simulink model "IEEE_39_IBR_Simplified"  (R2023b)
settings: Solver=FixedStepAuto  StartTime=0  StopTime=20  FixedStep=Ts  MaxStep=1/60  RelTol=1e-3  AbsTol=1e-2  EnableMultiTasking=on
PreLoadFcn:
  | NE39bus_data;
  | PSSMODEL=1;
  | LPSS=0;
  | WAPSS=0;
  | WAPSS2=0;
values from neighbouring files (symbols this model uses):
  Dt = 0    [SG_para.m]
  dw0_sm = 0    [SG_para.m]
  Emax = 1    [SG_para.m]
  Emin = 0.5    [SG_para.m]
  Fg = [0.1,0.1,0.1]    [SG_para.m]
  fn_sm = 60*ones(1,10)    [SG_para.m]
  H_sm = [5,3.03,3.58,2.86,2.6,3.48,2.64,2.43,3.45,4.2]*10    [SG_para.m]
  ia0_sm = 0.75*0    (= 0)    [SG_para.m]
  ib0_sm = 0.75*0    (= 0)    [SG_para.m]
  ic0_sm = 0.75*0    (= 0)    [SG_para.m]
  Kd_sm = 6*ones(1,10)    [SG_para.m]
  Ke = 200    [SG_para.m]
  Kg = [0.95,0.95,0.95]    [SG_para.m]
  Ks = 2    [SG_para.m]
  line = [     1	2	0.0035	0.0411	0.6987	0	100	345 ... (first row only)    [SG_para.m]
  p = 1    [SG_para.m]
  pha0_sm = -24.95*0    (= 0)    [SG_para.m]
  phb0_sm = -144.94*0    (= 0)    [SG_para.m]
  phc0_sm = 95.05*0    (= 0)    [SG_para.m]
  Pn_sm = [1000,1000,1000,1000,1000,1000,1000,1000,1000,1000]    [SG_para.m]
  Pref_sm = [1000 520.81 650 632 508 650 560 540 830 250]./Pn_sm    [SG_para.m]
  R = 1e-3    (= 0.001)    [SG_para.m]
  Rg = [0.05,0.05,0.05]    [SG_para.m]
  rs = 2.8544e-3    (= 0.0028544)    [SG_para.m]
  s = 1    [SG_para.m]
  s1 = 10    [SG_para.m]
  T1 = 0.05    [SG_para.m]
  T2 = 0.5    [SG_para.m]
  T3 = 0.5    [SG_para.m]
  Te = 0.05    [SG_para.m]
  Tfa = 3    [SG_para.m]
  Tfb = 10    [SG_para.m]
  Tg = [10,10,10]    [SG_para.m]
  theta0_sm = -94.3*0    (= 0)    [SG_para.m]
  Ts = 5e-5    (= 5e-05)    [SG_para.m]
  Ts1 = 0.18    [SG_para.m]
  Ts2 = 2    [SG_para.m]
  Ts3 = 5    [SG_para.m]
  Ts4 = 10    [SG_para.m]
  Ts5 = 15    [SG_para.m]
  Un_sm = [345,22,22,22,22,22,22,22,345,22]    [SG_para.m]
  Vmax = inf    [SG_para.m]
  Vmin = 0    [SG_para.m]
  Vref_sm = 1*ones(1,10)    [SG_para.m]
  xd = xd_t    (= 0.296)    [SG_para.m]
undefined symbols (not defined in the file or in its folder): D1, D11, Delta, Ka, Kf, Ta, Tf
libraries: spsThreePhaseVIMeasurementLib x41, spsThreePhaseFaultLib x39, spsThreePhaseSeriesRLCBranchLib x36, spsThreePhaseParallelRLCLoadLib x20, spsThreePhaseTransformerTwoWindingsLib x13, spsSimplifiedSynchronousMachinepuUnitsLib x10, spsLoadFlowBusLib x10, Inverter_based_Resources_IBRs x10, spsThreePhaseBreakerLib x2, spsSequenceAnalyzerLib x2, spsMultimeterLib x1, eePowerMeasurement x1
(part 3 of 5)

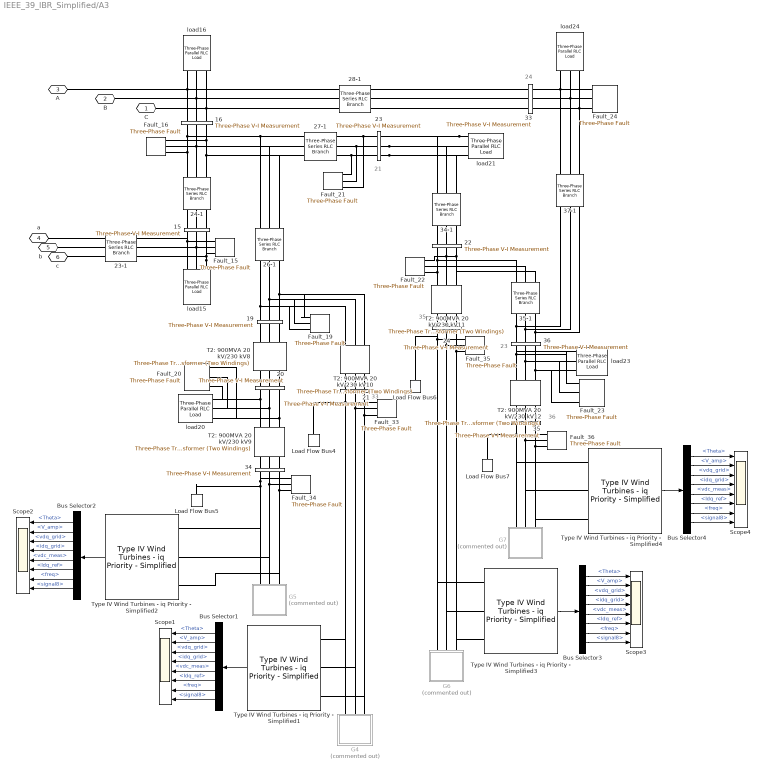
== system IEEE_39_IBR_Simplified/A3 ==
  note: 35
  note: 33
  note: 21
  note: 24
  note: 36
  note: 23
  15 : spsThreePhaseVIMeasurementLib/Three-Phase V-I Measurement  VoltageMeasurement=phase-to-phase  SetLabelV=on  LabelV=Vabc_15  Vpu=off  VpuLL=on  CurrentMeasurement=no  SetLabelI=on  LabelI=Iabc_B2  Ipu=off  Pbase=100e6  Vbase=Bus(15,2)*1e3  OutputType=Complex  PhasorSimulation=off  PSBequivalent=0
  16 : spsThreePhaseVIMeasurementLib/Three-Phase V-I Measurement  VoltageMeasurement=phase-to-phase  SetLabelV=on  LabelV=Vabc_16  Vpu=off  VpuLL=on  CurrentMeasurement=no  SetLabelI=on  LabelI=Iabc_B2  Ipu=off  Pbase=100e6  Vbase=Bus(16,2)*1e3  OutputType=Complex  PhasorSimulation=off  PSBequivalent=0
  19 : spsThreePhaseVIMeasurementLib/Three-Phase V-I Measurement  VoltageMeasurement=phase-to-phase  SetLabelV=on  LabelV=Vabc_19  Vpu=off  VpuLL=on  CurrentMeasurement=no  SetLabelI=on  LabelI=Iabc_B2  Ipu=off  Pbase=100e6  Vbase=Bus(19,2)*1e3  OutputType=Complex  PhasorSimulation=off  PSBequivalent=0
  20 : spsThreePhaseVIMeasurementLib/Three-Phase V-I Measurement  VoltageMeasurement=phase-to-phase  SetLabelV=on  LabelV=Vabc_20  Vpu=off  VpuLL=on  CurrentMeasurement=no  SetLabelI=on  LabelI=Iabc_B2  Ipu=off  Pbase=100e6  Vbase=Bus(20,2)*1e3  OutputType=Complex  PhasorSimulation=off  PSBequivalent=0
  21 : spsThreePhaseVIMeasurementLib/Three-Phase V-I Measurement  VoltageMeasurement=phase-to-phase  SetLabelV=on  LabelV=Vabc_33  Vpu=off  VpuLL=on  CurrentMeasurement=no  SetLabelI=on  LabelI=Iabc_B2  Ipu=off  Pbase=100e6  Vbase=Bus(33,2)*1e3  OutputType=Complex  PhasorSimulation=off  PSBequivalent=0
  22 : spsThreePhaseVIMeasurementLib/Three-Phase V-I Measurement  VoltageMeasurement=phase-to-phase  SetLabelV=on  LabelV=Vabc_22  Vpu=off  VpuLL=on  CurrentMeasurement=no  SetLabelI=on  LabelI=Iabc_B2  Ipu=off  Pbase=100e6  Vbase=Bus(22,2)*1e3  OutputType=Complex  PhasorSimulation=off  PSBequivalent=0
  23 : spsThreePhaseVIMeasurementLib/Three-Phase V-I Measurement  VoltageMeasurement=phase-to-phase  SetLabelV=on  LabelV=Vabc_21  Vpu=off  VpuLL=on  CurrentMeasurement=no  SetLabelI=on  LabelI=Iabc_B2  Ipu=off  Pbase=100e6  Vbase=Bus(21,2)*1e3  OutputType=Complex  PhasorSimulation=off  PSBequivalent=0
  23-1 : spsThreePhaseSeriesRLCBranchLib/Three-Phase Series RLC Branch  LConnTagsString=A|B|C  RConnTagsString=A|B|C  BranchType=RL  Resistance=line(23,3)  Inductance=line(23,4)  Capacitance=1e-6  Measurements=None
  24 : spsThreePhaseVIMeasurementLib/Three-Phase V-I Measurement  VoltageMeasurement=phase-to-phase  SetLabelV=on  LabelV=Vabc_35  Vpu=off  VpuLL=on  CurrentMeasurement=no  SetLabelI=on  LabelI=Iabc_B2  Ipu=off  Pbase=100e6  Vbase=Bus(35,2)*1e3  OutputType=Complex  PhasorSimulation=off  PSBequivalent=0
  24-1 : spsThreePhaseSeriesRLCBranchLib/Three-Phase Series RLC Branch  LConnTagsString=A|B|C  RConnTagsString=A|B|C  BranchType=RL  Resistance=line(24,3)  Inductance=line(24,4)  Capacitance=1e-6  Measurements=None
  26-1 : spsThreePhaseSeriesRLCBranchLib/Three-Phase Series RLC Branch  LConnTagsString=A|B|C  RConnTagsString=A|B|C  BranchType=RL  Resistance=line(26,3)  Inductance=line(26,4)  Capacitance=1e-6  Measurements=None
  27-1 : spsThreePhaseSeriesRLCBranchLib/Three-Phase Series RLC Branch  LConnTagsString=A|B|C  RConnTagsString=A|B|C  BranchType=RL  Resistance=line(27,3)  Inductance=line(27,4)  Capacitance=1e-6  Measurements=None
  28-1 : spsThreePhaseSeriesRLCBranchLib/Three-Phase Series RLC Branch  LConnTagsString=A|B|C  RConnTagsString=A|B|C  BranchType=RL  Resistance=line(28,3)  Inductance=line(28,4)  Capacitance=1e-6  Measurements=None
  33 : spsThreePhaseVIMeasurementLib/Three-Phase V-I Measurement  VoltageMeasurement=phase-to-phase  SetLabelV=on  LabelV=Vabc_24  Vpu=off  VpuLL=on  CurrentMeasurement=no  SetLabelI=on  LabelI=Iabc_B2  Ipu=off  Pbase=100e6  Vbase=Bus(24,2)*1e3  OutputType=Complex  PhasorSimulation=off  PSBequivalent=0
  34 : spsThreePhaseVIMeasurementLib/Three-Phase V-I Measurement  VoltageMeasurement=phase-to-phase  SetLabelV=on  LabelV=Vabc_34  Vpu=off  VpuLL=on  CurrentMeasurement=no  SetLabelI=on  LabelI=Iabc_B2  Ipu=off  Pbase=100e6  Vbase=Bus(34,2)*1e3  OutputType=Complex  PhasorSimulation=off  PSBequivalent=0
  34-1 : spsThreePhaseSeriesRLCBranchLib/Three-Phase Series RLC Branch  LConnTagsString=A|B|C  RConnTagsString=A|B|C  BranchType=RL  Resistance=line(34,3)  Inductance=line(34,4)  Capacitance=1e-6  Measurements=None
  35 : spsThreePhaseVIMeasurementLib/Three-Phase V-I Measurement  VoltageMeasurement=phase-to-phase  SetLabelV=on  LabelV=Vabc_36  Vpu=off  VpuLL=on  CurrentMeasurement=no  SetLabelI=on  LabelI=Iabc_B2  Ipu=off  Pbase=100e6  Vbase=Bus(36,2)*1e3  OutputType=Complex  PhasorSimulation=off  PSBequivalent=0
  35-1 : spsThreePhaseSeriesRLCBranchLib/Three-Phase Series RLC Branch  LConnTagsString=A|B|C  RConnTagsString=A|B|C  BranchType=RL  Resistance=line(35,3)  Inductance=line(35,4)  Capacitance=1e-6  Measurements=None
  36 : spsThreePhaseVIMeasurementLib/Three-Phase V-I Measurement  VoltageMeasurement=phase-to-phase  SetLabelV=on  LabelV=Vabc_23  Vpu=off  VpuLL=on  CurrentMeasurement=no  SetLabelI=on  LabelI=Iabc_B2  Ipu=off  Pbase=100e6  Vbase=Bus(23,2)*1e3  OutputType=Complex  PhasorSimulation=off  PSBequivalent=0
  37-1 : spsThreePhaseSeriesRLCBranchLib/Three-Phase Series RLC Branch  LConnTagsString=A|B|C  RConnTagsString=A|B|C  BranchType=RL  Resistance=line(37,3)  Inductance=line(37,4)  Capacitance=1e-6  Measurements=None
  Bus Selector{1..4} (4 alike) : BusSelector  OutputSignals=Theta,V_amp,vdq_grid,idq_grid,vdc_meas,Idq_ref,freq,signal8
  Fault_15 : spsThreePhaseFaultLib/Three-Phase Fault  InitialStates=0  FaultA=on  FaultB=on  FaultC=on  GroundFault=on  SwitchTimes="[t(15)+1/60  t(15)+5/60]"  External=off  SwitchStatus=NaN  FaultResistance=0.001  GroundResistance=0.01  SnubberResistance=1e6  SnubberCapacitance=inf  Measurements=Fault voltages and currents
  Fault_16 : spsThreePhaseFaultLib/Three-Phase Fault  InitialStates=0  FaultA=on  FaultB=on  FaultC=on  GroundFault=on  SwitchTimes="[t(16)+1/60  t(16)+5/60]"  External=off  SwitchStatus=NaN  FaultResistance=0.001  GroundResistance=0.01  SnubberResistance=1e6  SnubberCapacitance=inf  Measurements=Fault voltages and currents
  Fault_19 : spsThreePhaseFaultLib/Three-Phase Fault  InitialStates=0  FaultA=on  FaultB=on  FaultC=on  GroundFault=on  SwitchTimes="[t(19)+1/60  t(19)+5/60]"  External=off  SwitchStatus=NaN  FaultResistance=0.001  GroundResistance=0.01  SnubberResistance=1e6  SnubberCapacitance=inf  Measurements=Fault voltages and currents
  Fault_20 : spsThreePhaseFaultLib/Three-Phase Fault  InitialStates=0  FaultA=on  FaultB=on  FaultC=on  GroundFault=on  SwitchTimes="[t(20)+1/60  t(20)+5/60]"  External=off  SwitchStatus=NaN  FaultResistance=0.001  GroundResistance=0.01  SnubberResistance=1e6  SnubberCapacitance=inf  Measurements=Fault voltages and currents
  Fault_21 : spsThreePhaseFaultLib/Three-Phase Fault  InitialStates=0  FaultA=on  FaultB=on  FaultC=on  GroundFault=on  SwitchTimes="[t(21)+1/60  t(21)+5/60]"  External=off  SwitchStatus=NaN  FaultResistance=0.001  GroundResistance=0.01  SnubberResistance=1e6  SnubberCapacitance=inf  Measurements=Fault voltages and currents
  Fault_22 : spsThreePhaseFaultLib/Three-Phase Fault  InitialStates=0  FaultA=on  FaultB=on  FaultC=on  GroundFault=on  SwitchTimes="[t(22)+1/60  t(22)+5/60]"  External=off  SwitchStatus=NaN  FaultResistance=0.001  GroundResistance=0.01  SnubberResistance=1e6  SnubberCapacitance=inf  Measurements=Fault voltages and currents
  Fault_23 : spsThreePhaseFaultLib/Three-Phase Fault  InitialStates=0  FaultA=on  FaultB=on  FaultC=on  GroundFault=on  SwitchTimes="[t(23)+1/60  t(23)+5/60]"  External=off  SwitchStatus=NaN  FaultResistance=0.001  GroundResistance=0.01  SnubberResistance=1e6  SnubberCapacitance=inf  Measurements=Fault voltages and currents
  Fault_24 : spsThreePhaseFaultLib/Three-Phase Fault  InitialStates=0  FaultA=on  FaultB=on  FaultC=on  GroundFault=on  SwitchTimes="[t(24)+1/60  t(24)+5/60]"  External=off  SwitchStatus=NaN  FaultResistance=0.001  GroundResistance=0.01  SnubberResistance=1e6  SnubberCapacitance=inf  Measurements=Fault voltages and currents
  Fault_33 : spsThreePhaseFaultLib/Three-Phase Fault  InitialStates=0  FaultA=on  FaultB=on  FaultC=on  GroundFault=on  SwitchTimes="[t(33)+1/60  t(33)+5/60]"  External=off  SwitchStatus=NaN  FaultResistance=0.001  GroundResistance=0.01  SnubberResistance=1e6  SnubberCapacitance=inf  Measurements=Fault voltages and currents
  Fault_34 : spsThreePhaseFaultLib/Three-Phase Fault  InitialStates=0  FaultA=on  FaultB=on  FaultC=on  GroundFault=on  SwitchTimes="[t(34)+1/60  t(34)+5/60]"  External=off  SwitchStatus=NaN  FaultResistance=0.001  GroundResistance=0.01  SnubberResistance=1e6  SnubberCapacitance=inf  Measurements=Fault voltages and currents
  Fault_35 : spsThreePhaseFaultLib/Three-Phase Fault  InitialStates=0  FaultA=on  FaultB=on  FaultC=on  GroundFault=on  SwitchTimes="[t(35)+1/60  t(35)+5/60]"  External=off  SwitchStatus=NaN  FaultResistance=0.001  GroundResistance=0.01  SnubberResistance=1e6  SnubberCapacitance=inf  Measurements=Fault voltages and currents
  Fault_36 : spsThreePhaseFaultLib/Three-Phase Fault  InitialStates=0  FaultA=on  FaultB=on  FaultC=on  GroundFault=on  SwitchTimes="[t(36)+1/60  t(36)+5/60]"  External=off  SwitchStatus=NaN  FaultResistance=0.001  GroundResistance=0.01  SnubberResistance=1e6  SnubberCapacitance=inf  Measurements=Fault voltages and currents
  G4 : Subsystem  Commented=on
  G5 : Subsystem  Commented=on
  G6 : Subsystem  Commented=on
  G7 : Subsystem  Commented=on
  Load Flow Bus4 : spsLoadFlowBusLib/Load Flow Bus  LConnTagsString=a  Phases=single  Connectors=on one side  ID=Bus33  Vbase=22e3  Vref=0.9972  Vangle=0  VLF=0.9972  VLFb=1  VLFc=1  angleLF=4.423  angleLFb=0  angleLFc=0
      settings: AttributesFormatString=%<ID>\n%<Vbase>V\n%<VLF>pu\n%<angleLF>deg.
  Load Flow Bus5 : spsLoadFlowBusLib/Load Flow Bus  LConnTagsString=a  Phases=single  Connectors=on one side  ID=Bus34  Vbase=22e3  Vref=1.0123  Vangle=0  VLF=1.012  VLFb=1  VLFc=1  angleLF=3.398  angleLFb=0  angleLFc=0
      settings: AttributesFormatString=%<ID>\n%<Vbase>V\n%<VLF>pu\n%<angleLF>deg.
  Load Flow Bus6 : spsLoadFlowBusLib/Load Flow Bus  LConnTagsString=a  Phases=single  Connectors=on one side  ID=Bus35  Vbase=22e3  Vref=1.0493  Vangle=0  VLF=1.049  VLFb=1  VLFc=1  angleLF=5.698  angleLFb=0  angleLFc=0
      settings: AttributesFormatString=%<ID>\n%<Vbase>V\n%<VLF>pu\n%<angleLF>deg.
  Load Flow Bus7 : spsLoadFlowBusLib/Load Flow Bus  LConnTagsString=a  Phases=single  Connectors=on one side  ID=Bus36  Vbase=22e3  Vref=1.0635  Vangle=0  VLF=1.063  VLFb=1  VLFc=1  angleLF=8.494  angleLFb=0  angleLFc=0
      settings: AttributesFormatString=%<ID>\n%<Vbase>V\n%<VLF>pu\n%<angleLF>deg.
  Scope{1..4} (4 alike) : Scope  NumInputPorts=8
  T2: 900MVA 20 kV/230 kV10 : spsThreePhaseTransformerTwoWindingsLib/Three-Phase Transformer (Two Windings)  Winding1Connection=Delta (D1)  Winding2Connection=Yg  CoreType=Three single-phase transformers  SetSaturation=off  Hysteresis=off  DataFile='hysteresis'  SetInitialFlux=off  Measurements=None  UNITS=pu  NominalPower=[ 1000e6 60 ]  Winding1="[ 22e3*1.0   0.00035*s  0]"  Winding2="[ 345e3*1.0  0.00035*s  0.0142*s]"  Rm=500  Lm=500  L0=0.5  Saturation="[ 0,0  ;  0.005,1.2  ;  1.0,1.4 ]"  InitialFluxes=[ 0.8 , -0.8 , 0.7 ]  BreakLoop=off  DiscreteSolver=Trapezoidal iterative  DataType=off  TransfoNumber=0
  T2: 900MVA 20 kV/230 kV11 : spsThreePhaseTransformerTwoWindingsLib/Three-Phase Transformer (Two Windings)  Winding1Connection=Delta (D1)  Winding2Connection=Yg  CoreType=Three single-phase transformers  SetSaturation=off  Hysteresis=off  DataFile='hysteresis'  SetInitialFlux=off  Measurements=None  UNITS=pu  NominalPower=[ 1000e6 60 ]  Winding1="[ 22e3*1.0  1e-6  0]"  Winding2="[ 345e3*1.0  1e-6  0.0143*s]"  Rm=500  Lm=500  L0=0.5  Saturation="[ 0,0  ;  0.005,1.2  ;  1.0,1.4 ]"  InitialFluxes=[ 0.8 , -0.8 , 0.7 ]  BreakLoop=off  DiscreteSolver=Trapezoidal iterative  DataType=off  TransfoNumber=0
  T2: 900MVA 20 kV/230 kV12 : spsThreePhaseTransformerTwoWindingsLib/Three-Phase Transformer (Two Windings)  Winding1Connection=Delta (D1)  Winding2Connection=Yg  CoreType=Three single-phase transformers  SetSaturation=off  Hysteresis=off  DataFile='hysteresis'  SetInitialFlux=off  Measurements=None  UNITS=pu  NominalPower=[ 1000e6 60 ]  Winding1="[ 22e3    0.00025*s  0.0]"  Winding2="[ 345e3    0.00025*s  0.0272*s]"  Rm=500  Lm=500  L0=0.5  Saturation="[ 0,0  ;  0.005,1.2  ;  1.0,1.4 ]"  InitialFluxes=[ 0.8 , -0.8 , 0.7 ]  BreakLoop=off  DiscreteSolver=Trapezoidal iterative  DataType=off  TransfoNumber=0
  T2: 900MVA 20 kV/230 kV8 : spsThreePhaseTransformerTwoWindingsLib/Three-Phase Transformer (Two Windings)  Winding1Connection=Y  Winding2Connection=Y  CoreType=Three single-phase transformers  SetSaturation=off  Hysteresis=off  DataFile='hysteresis'  SetInitialFlux=off  Measurements=None  UNITS=pu  NominalPower=[ 1000e6 60 ]  Winding1="[ 345e3*1.0  0.00035*s   0]"  Winding2="[ 345e3*1.00 0.00035*s  0.0138*s1]"  Rm=500  Lm=500  L0=0.5  Saturation="[ 0,0  ;  0.005,1.2  ;  1.0,1.4 ]"  InitialFluxes=[ 0.8 , -0.8 , 0.7 ]  BreakLoop=off  DiscreteSolver=Trapezoidal iterative  DataType=off  TransfoNumber=0
  T2: 900MVA 20 kV/230 kV9 : spsThreePhaseTransformerTwoWindingsLib/Three-Phase Transformer (Two Windings)  Winding1Connection=Delta (D1)  Winding2Connection=Yg  CoreType=Three single-phase transformers  SetSaturation=off  Hysteresis=off  DataFile='hysteresis'  SetInitialFlux=off  Measurements=None  UNITS=pu  NominalPower=[ 1000e6 60 ]  Winding1="[ 22e3*1.00 0.00045*s  0]"  Winding2="[ 345e3*1  0.00045*s  0.0180*s]"  Rm=500  Lm=500  L0=0.5  Saturation="[ 0,0  ;  0.005,1.2  ;  1.0,1.4 ]"  InitialFluxes=[ 0.8 , -0.8 , 0.7 ]  BreakLoop=off  DiscreteSolver=Trapezoidal iterative  DataType=off  TransfoNumber=0
  Type IV Wind Turbines - iq Priority - Simplified1 : Inverter_based_Resources_IBRs/Inverter-based Resources (IBRs)/Type IV Wind Turbines - iq Priority - Simplified  Num_WTs=1  Wind_Speed_WT=15  Q_ref_pu_WT=0  Transformer_P_f="[1000e6  60]"  Transformer_V1_R1_L1=[22e3 , 0.025/30 , 0.025]  DC_Power=1000e6*0.4918
  Type IV Wind Turbines - iq Priority - Simplified2 : Inverter_based_Resources_IBRs/Inverter-based Resources (IBRs)/Type IV Wind Turbines - iq Priority - Simplified  Num_WTs=1  Wind_Speed_WT=15  Q_ref_pu_WT=0  Transformer_P_f="[1000e6  60]"  Transformer_V1_R1_L1=[22e3 , 0.025/30 , 0.025]  DC_Power=1000e6*0.3682
  Type IV Wind Turbines - iq Priority - Simplified3 : Inverter_based_Resources_IBRs/Inverter-based Resources (IBRs)/Type IV Wind Turbines - iq Priority - Simplified  Num_WTs=1  Wind_Speed_WT=15  Q_ref_pu_WT=0  Transformer_P_f="[1000e6  60]"  Transformer_V1_R1_L1=[22e3 , 0.025/30 , 0.025]  DC_Power=1000e6*0.5094
  Type IV Wind Turbines - iq Priority - Simplified4 : Inverter_based_Resources_IBRs/Inverter-based Resources (IBRs)/Type IV Wind Turbines - iq Priority - Simplified  Num_WTs=1  Wind_Speed_WT=15  Q_ref_pu_WT=0  Transformer_P_f="[1000e6  60]"  Transformer_V1_R1_L1=[22e3 , 0.025/30 , 0.025]  DC_Power=1000e6*0.4199
  load15 : spsThreePhaseParallelRLCLoadLib/Three-Phase Parallel RLC Load  LConnTagsString=A|B|C  Configuration=Y (grounded)  NominalVoltage=(345000)*0.969586  Vabc=[1e3 1e3 1e3]  Vabcp=[1e3 1e3 1e3]  NominalFrequency=60  UnbalancedPower=off  ActivePower=320e6  InductivePower=153e6  CapacitivePower=0  Pabc=[10e3 9e3 11e3]  QLabc=[100 90 110]  QCabc=[100 90 110]  Pabcp=[10e3 9e3 11e3]  QLabcp=[100 90 110]  QCabcp=[100 90 110]  Measurements=None  LoadType=constant PQ
  load16 : spsThreePhaseParallelRLCLoadLib/Three-Phase Parallel RLC Load  LConnTagsString=A|B|C  Configuration=Y (grounded)  NominalVoltage=(345000)*0.988678  Vabc=[1e3 1e3 1e3]  Vabcp=[1e3 1e3 1e3]  NominalFrequency=60  UnbalancedPower=off  ActivePower=329e6  InductivePower=32.3e6  CapacitivePower=0  Pabc=[10e3 9e3 11e3]  QLabc=[100 90 110]  QCabc=[100 90 110]  Pabcp=[10e3 9e3 11e3]  QLabcp=[100 90 110]  QCabcp=[100 90 110]  Measurements=None  LoadType=constant PQ
  load20 : spsThreePhaseParallelRLCLoadLib/Three-Phase Parallel RLC Load  LConnTagsString=A|B|C  Configuration=Y (grounded)  NominalVoltage=(345000)*0.987086  Vabc=[1e3 1e3 1e3]  Vabcp=[1e3 1e3 1e3]  NominalFrequency=60  UnbalancedPower=off  ActivePower=628e6  InductivePower=103e6  CapacitivePower=0  Pabc=[10e3 9e3 11e3]  QLabc=[100 90 110]  QCabc=[100 90 110]  Pabcp=[10e3 9e3 11e3]  QLabcp=[100 90 110]  QCabcp=[100 90 110]  Measurements=None  LoadType=constant PQ
  load21 : spsThreePhaseParallelRLCLoadLib/Three-Phase Parallel RLC Load  LConnTagsString=A|B|C  Configuration=Y (grounded)  NominalVoltage=(345000)*0.995503  Vabc=[1e3 1e3 1e3]  Vabcp=[1e3 1e3 1e3]  NominalFrequency=60  UnbalancedPower=off  ActivePower=274e6  InductivePower=115e6  CapacitivePower=0  Pabc=[10e3 9e3 11e3]  QLabc=[100 90 110]  QCabc=[100 90 110]  Pabcp=[10e3 9e3 11e3]  QLabcp=[100 90 110]  QCabcp=[100 90 110]  Measurements=None  LoadType=constant PQ
  load23 : spsThreePhaseParallelRLCLoadLib/Three-Phase Parallel RLC Load  LConnTagsString=A|B|C  Configuration=Y (grounded)  NominalVoltage=(345000)*1.02041  Vabc=[1e3 1e3 1e3]  Vabcp=[1e3 1e3 1e3]  NominalFrequency=60  UnbalancedPower=off  ActivePower=247.5e6  InductivePower=84.6e6  CapacitivePower=0  Pabc=[10e3 9e3 11e3]  QLabc=[100 90 110]  QCabc=[100 90 110]  Pabcp=[10e3 9e3 11e3]  QLabcp=[100 90 110]  QCabcp=[100 90 110]  Measurements=None  LoadType=constant PQ
  load24 : spsThreePhaseParallelRLCLoadLib/Three-Phase Parallel RLC Load  LConnTagsString=A|B|C  Configuration=Y (grounded)  NominalVoltage=(345000)*0.996934  Vabc=[1e3 1e3 1e3]  Vabcp=[1e3 1e3 1e3]  NominalFrequency=60  UnbalancedPower=off  ActivePower=308.6e6  InductivePower=0  CapacitivePower=92e6  Pabc=[10e3 9e3 11e3]  QLabc=[100 90 110]  QCabc=[100 90 110]  Pabcp=[10e3 9e3 11e3]  QLabcp=[100 90 110]  QCabcp=[100 90 110]  Measurements=None  LoadType=constant PQ
  C : PMIOPort  Side=Left
  B : PMIOPort  Port=2  Side=Left
  A : PMIOPort  Port=3  Side=Left
  a : PMIOPort  Port=4  Side=Right
  b : PMIOPort  Port=5  Side=Right
  c : PMIOPort  Port=6  Side=Right
  wires:
  Bus Selector1/5 -> Scope1/5  "<vdc_meas>"
  Bus Selector1/4 -> Scope1/4  "<idq_grid>"
  Bus Selector1/7 -> Scope1/7  "<freq>"
  Bus Selector1/8 -> Scope1/8  "<signal8>"
  Type IV Wind Turbines - iq Priority - Simplified1/1 -> Bus Selector1/1
  Bus Selector1/1 -> Scope1/1  "<Theta>"
  Bus Selector1/6 -> Scope1/6  "<Idq_ref>"
  Bus Selector1/3 -> Scope1/3  "<vdq_grid>"
  Bus Selector1/2 -> Scope1/2  "<V_amp>"
  Bus Selector2/5 -> Scope2/5  "<vdc_meas>"
  Bus Selector2/4 -> Scope2/4  "<idq_grid>"
  Bus Selector2/7 -> Scope2/7  "<freq>"
  Bus Selector2/8 -> Scope2/8  "<signal8>"
  Type IV Wind Turbines - iq Priority - Simplified2/1 -> Bus Selector2/1
  Bus Selector2/1 -> Scope2/1  "<Theta>"
  Bus Selector2/6 -> Scope2/6  "<Idq_ref>"
  Bus Selector2/3 -> Scope2/3  "<vdq_grid>"
  Bus Selector2/2 -> Scope2/2  "<V_amp>"
  Bus Selector3/5 -> Scope3/5  "<vdc_meas>"
  Bus Selector3/4 -> Scope3/4  "<idq_grid>"
  Bus Selector3/7 -> Scope3/7  "<freq>"
  Bus Selector3/8 -> Scope3/8  "<signal8>"
  Type IV Wind Turbines - iq Priority - Simplified3/1 -> Bus Selector3/1
  Bus Selector3/1 -> Scope3/1  "<Theta>"
  Bus Selector3/6 -> Scope3/6  "<Idq_ref>"
  Bus Selector3/3 -> Scope3/3  "<vdq_grid>"
  Bus Selector3/2 -> Scope3/2  "<V_amp>"
  Type IV Wind Turbines - iq Priority - Simplified4/1 -> Bus Selector4/1
  Bus Selector4/5 -> Scope4/5  "<vdc_meas>"
  Bus Selector4/3 -> Scope4/3  "<vdq_grid>"
  Bus Selector4/2 -> Scope4/2  "<V_amp>"
  Bus Selector4/8 -> Scope4/8  "<signal8>"
  Bus Selector4/6 -> Scope4/6  "<Idq_ref>"
  Bus Selector4/1 -> Scope4/1  "<Theta>"
  Bus Selector4/7 -> Scope4/7  "<freq>"
  Bus Selector4/4 -> Scope4/4  "<idq_grid>"
  connections:
  T2: 900MVA 20 kV/230 kV10/LConn1 -- 21/RConn1
  34-1/RConn3 -- 22/LConn3
  Fault_15/LConn2 -- 23-1/LConn2 -- load15/LConn2 -- 15/RConn2
  T2: 900MVA 20 kV/230 kV9/RConn1 -- Fault_20/LConn1 -- load20/LConn1 -- 20/RConn1
  T2: 900MVA 20 kV/230 kV12/LConn2 -- 35/LConn2
  Fault_16/LConn1 -- 24-1/LConn1 -- 16/LConn1 -- 26-1/LConn1 -- 27-1/RConn1
  T2: 900MVA 20 kV/230 kV12/LConn3 -- 35/LConn3
  22/RConn2 -- 35-1/LConn2 -- Fault_22/LConn2 -- T2: 900MVA 20 kV/230 kV11/RConn2
  T2: 900MVA 20 kV/230 kV8/LConn3 -- 19/RConn3
  Fault_19/LConn3 -- T2: 900MVA 20 kV/230 kV10/RConn1 -- 26-1/RConn1 -- 19/LConn1
  36/LConn1 -- 35-1/RConn1 -- 37-1/RConn1
  Fault_15/LConn1 -- 23-1/LConn1 -- load15/LConn1 -- 15/RConn1
  T2: 900MVA 20 kV/230 kV8/RConn2 -- 20/LConn2
  T2: 900MVA 20 kV/230 kV12/RConn2 -- Fault_23/LConn2 -- load23/LConn2 -- 36/RConn2
  Fault_24/LConn1 -- 37-1/LConn1 -- load24/LConn1 -- 33/RConn1
  Fault_16/LConn2 -- 24-1/LConn2 -- 26-1/LConn2 -- 27-1/RConn2 -- 16/LConn2
  load21/LConn1 -- 34-1/LConn1 -- 23/RConn1
  Fault_34/LConn3 -- Type IV Wind Turbines - iq Priority - Simplified2/LConn3 -- G5/LConn3 -- 34/RConn3
  T2: 900MVA 20 kV/230 kV11/RConn1 -- Fault_22/LConn1 -- 35-1/LConn1 -- 22/RConn1
  34-1/RConn2 -- 22/LConn2
  load16/LConn3 -- C/RConn1 -- 28-1/RConn3 -- 16/RConn3
  36/LConn3 -- 35-1/RConn3 -- 37-1/RConn3
  21/LConn2 -- Type IV Wind Turbines - iq Priority - Simplified1/LConn2 -- G4/LConn2 -- Fault_33/LConn2
  T2: 900MVA 20 kV/230 kV8/RConn1 -- 20/LConn1
  Fault_24/LConn3 -- 37-1/LConn3 -- load24/LConn3 -- 33/RConn3
  21/LConn1 -- G4/LConn1 -- Type IV Wind Turbines - iq Priority - Simplified1/LConn1 -- Fault_33/LConn1 -- Load Flow Bus4/LConn1
  Fault_19/LConn1 -- T2: 900MVA 20 kV/230 kV10/RConn3 -- 26-1/RConn3 -- 19/LConn3
  T2: 900MVA 20 kV/230 kV12/LConn1 -- 35/LConn1
  load15/LConn3 -- 23-1/LConn3 -- Fault_15/LConn3 -- 15/RConn3
  Fault_24/LConn2 -- 37-1/LConn2 -- load24/LConn2 -- 33/RConn2
  36/LConn2 -- 35-1/RConn2 -- 37-1/RConn2
  T2: 900MVA 20 kV/230 kV11/LConn3 -- 24/LConn3
  23-1/RConn2 -- b/RConn1
  T2: 900MVA 20 kV/230 kV8/LConn2 -- 19/RConn2
  35/RConn1 -- Type IV Wind Turbines - iq Priority - Simplified4/LConn1 -- G7/LConn1 -- Fault_36/LConn1 -- Load Flow Bus7/LConn1
  Load Flow Bus5/LConn1 -- Type IV Wind Turbines - iq Priority - Simplified2/LConn1 -- G5/LConn1 -- Fault_34/LConn1 -- 34/RConn1
  35/RConn3 -- Type IV Wind Turbines - iq Priority - Simplified4/LConn3 -- G7/LConn3 -- Fault_36/LConn3
  34/LConn3 -- T2: 900MVA 20 kV/230 kV9/LConn3
  24-1/LConn3 -- 26-1/LConn3 -- 27-1/RConn3 -- Fault_16/LConn3 -- 16/LConn3
  T2: 900MVA 20 kV/230 kV12/RConn1 -- Fault_23/LConn1 -- load23/LConn1 -- 36/RConn1
  34-1/RConn1 -- 22/LConn1
  35/RConn2 -- Type IV Wind Turbines - iq Priority - Simplified4/LConn2 -- G7/LConn2 -- Fault_36/LConn2
  23/RConn2 -- 34-1/LConn2 -- load21/LConn2
  28-1/LConn2 -- 33/LConn2
  28-1/LConn3 -- 33/LConn3
  28-1/LConn1 -- 33/LConn1
  T2: 900MVA 20 kV/230 kV11/LConn2 -- 24/LConn2
  Fault_21/LConn2 -- 27-1/LConn2 -- 23/LConn2
  35-1/LConn3 -- T2: 900MVA 20 kV/230 kV11/RConn3 -- Fault_22/LConn3 -- 22/RConn3
  21/LConn3 -- G4/LConn3 -- Type IV Wind Turbines - iq Priority - Simplified1/LConn3 -- Fault_33/LConn3
  16/RConn1 -- A/RConn1 -- 28-1/RConn1 -- load16/LConn1
  16/RConn2 -- B/RConn1 -- 28-1/RConn2 -- load16/LConn2
  T2: 900MVA 20 kV/230 kV10/LConn3 -- 21/RConn3
  T2: 900MVA 20 kV/230 kV9/RConn3 -- Fault_20/LConn3 -- load20/LConn3 -- 20/RConn3
  Fault_21/LConn3 -- 27-1/LConn3 -- 23/LConn3
  Fault_21/LConn1 -- 27-1/LConn1 -- 23/LConn1
  Fault_19/LConn2 -- T2: 900MVA 20 kV/230 kV10/RConn2 -- 26-1/RConn2 -- 19/LConn2
  T2: 900MVA 20 kV/230 kV12/RConn3 -- Fault_23/LConn3 -- load23/LConn3 -- 36/RConn3
  24-1/RConn1 -- 15/LConn1
  24-1/RConn3 -- 15/LConn3
  Fault_34/LConn2 -- Type IV Wind Turbines - iq Priority - Simplified2/LConn2 -- G5/LConn2 -- 34/RConn2
  24-1/RConn2 -- 15/LConn2
  T2: 900MVA 20 kV/230 kV8/LConn1 -- 19/RConn1
  24/RConn2 -- Type IV Wind Turbines - iq Priority - Simplified3/LConn2 -- G6/LConn2 -- Fault_35/LConn2
  24/RConn1 -- Type IV Wind Turbines - iq Priority - Simplified3/LConn1 -- G6/LConn1 -- Fault_35/LConn1 -- Load Flow Bus6/LConn1
  24/RConn3 -- Type IV Wind Turbines - iq Priority - Simplified3/LConn3 -- G6/LConn3 -- Fault_35/LConn3
  23/RConn3 -- 34-1/LConn3 -- load21/LConn3
  T2: 900MVA 20 kV/230 kV9/RConn2 -- Fault_20/LConn2 -- load20/LConn2 -- 20/RConn2
  34/LConn2 -- T2: 900MVA 20 kV/230 kV9/LConn2
  34/LConn1 -- T2: 900MVA 20 kV/230 kV9/LConn1
  24/LConn1 -- T2: 900MVA 20 kV/230 kV11/LConn1
  T2: 900MVA 20 kV/230 kV8/RConn3 -- 20/LConn3
  T2: 900MVA 20 kV/230 kV10/LConn2 -- 21/RConn2
  23-1/RConn1 -- a/RConn1
  23-1/RConn3 -- c/RConn1

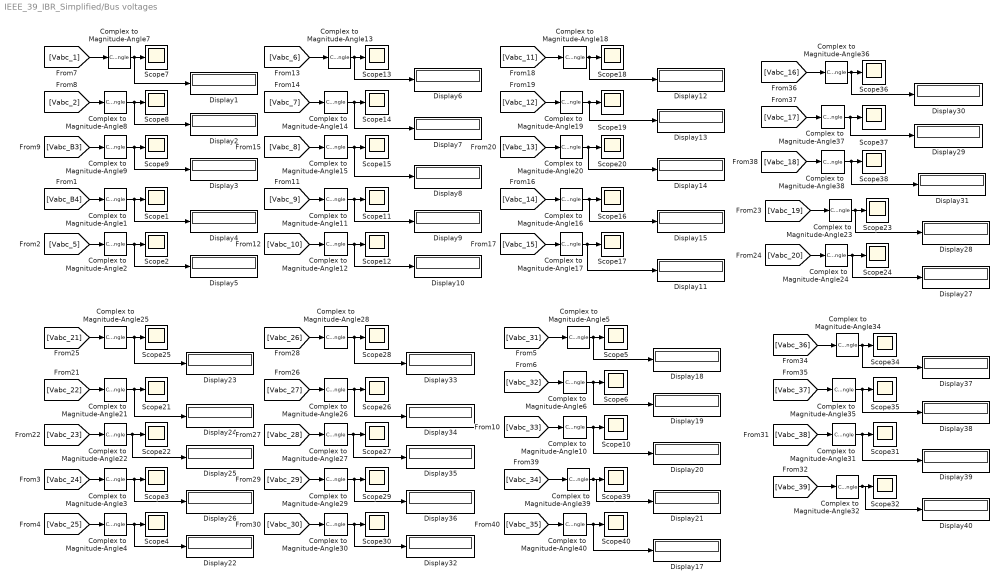
== system IEEE_39_IBR_Simplified/Bus voltages ==
  Complex to Magnitude-Angle{1..32,34..40} (39 alike) : ComplexToMagnitudeAngle  Output=Magnitude
  Display{1..15,17..40} (39 alike) : Display
  Scope{1..32,34..40} (39 alike) : Scope
  wires:
  [Vabc_1] -> Complex to Magnitude-Angle7/1
  Complex to Magnitude-Angle7/1 -> Display1/1, Scope7/1
  [Vabc_2] -> Complex to Magnitude-Angle8/1
  Complex to Magnitude-Angle8/1 -> Display2/1, Scope8/1
  [Vabc_B3] -> Complex to Magnitude-Angle9/1
  Complex to Magnitude-Angle9/1 -> Display3/1, Scope9/1
  [Vabc_B4] -> Complex to Magnitude-Angle1/1
  Complex to Magnitude-Angle1/1 -> Display4/1, Scope1/1
  [Vabc_5] -> Complex to Magnitude-Angle2/1
  Complex to Magnitude-Angle2/1 -> Display5/1, Scope2/1
  [Vabc_31] -> Complex to Magnitude-Angle5/1
  [Vabc_32] -> Complex to Magnitude-Angle6/1
  [Vabc_33] -> Complex to Magnitude-Angle10/1
  [Vabc_24] -> Complex to Magnitude-Angle3/1
  [Vabc_25] -> Complex to Magnitude-Angle4/1
  [Vabc_6] -> Complex to Magnitude-Angle13/1
  [Vabc_7] -> Complex to Magnitude-Angle14/1
  [Vabc_8] -> Complex to Magnitude-Angle15/1
  [Vabc_9] -> Complex to Magnitude-Angle11/1
  [Vabc_10] -> Complex to Magnitude-Angle12/1
  [Vabc_11] -> Complex to Magnitude-Angle18/1
  Complex to Magnitude-Angle18/1 -> Display12/1, Scope18/1
  [Vabc_12] -> Complex to Magnitude-Angle19/1
  [Vabc_13] -> Complex to Magnitude-Angle20/1
  Complex to Magnitude-Angle20/1 -> Display14/1, Scope20/1
  [Vabc_14] -> Complex to Magnitude-Angle16/1
  Complex to Magnitude-Angle16/1 -> Display15/1, Scope16/1
  [Vabc_15] -> Complex to Magnitude-Angle17/1
  Complex to Magnitude-Angle17/1 -> Display11/1, Scope17/1
  [Vabc_19] -> Complex to Magnitude-Angle23/1
  [Vabc_20] -> Complex to Magnitude-Angle24/1
  [Vabc_21] -> Complex to Magnitude-Angle25/1
  [Vabc_22] -> Complex to Magnitude-Angle21/1
  [Vabc_23] -> Complex to Magnitude-Angle22/1
  Complex to Magnitude-Angle13/1 -> Display6/1, Scope13/1
  Complex to Magnitude-Angle14/1 -> Display7/1, Scope14/1
  Complex to Magnitude-Angle15/1 -> Display8/1, Scope15/1
  Complex to Magnitude-Angle11/1 -> Display9/1, Scope11/1
  Complex to Magnitude-Angle12/1 -> Display10/1, Scope12/1
  Complex to Magnitude-Angle19/1 -> Display13/1, Scope19/1
  [Vabc_16] -> Complex to Magnitude-Angle36/1
  [Vabc_17] -> Complex to Magnitude-Angle37/1
  [Vabc_18] -> Complex to Magnitude-Angle38/1
  Complex to Magnitude-Angle38/1 -> Display31/1, Scope38/1
  [Vabc_34] -> Complex to Magnitude-Angle39/1
  [Vabc_35] -> Complex to Magnitude-Angle40/1
  Complex to Magnitude-Angle5/1 -> Display18/1, Scope5/1
  Complex to Magnitude-Angle10/1 -> Display20/1, Scope10/1
  Complex to Magnitude-Angle39/1 -> Display21/1, Scope39/1
  Complex to Magnitude-Angle40/1 -> Display17/1, Scope40/1
  Complex to Magnitude-Angle6/1 -> Display19/1, Scope6/1
  Complex to Magnitude-Angle25/1 -> Display23/1, Scope25/1
  Complex to Magnitude-Angle22/1 -> Display25/1, Scope22/1
  Complex to Magnitude-Angle3/1 -> Display26/1, Scope3/1
  Complex to Magnitude-Angle4/1 -> Display22/1, Scope4/1
  Complex to Magnitude-Angle21/1 -> Display24/1, Scope21/1
  Complex to Magnitude-Angle23/1 -> Display28/1, Scope23/1
  Complex to Magnitude-Angle24/1 -> Display27/1, Scope24/1
  Complex to Magnitude-Angle36/1 -> Display30/1, Scope36/1
  Complex to Magnitude-Angle37/1 -> Display29/1, Scope37/1
  [Vabc_29] -> Complex to Magnitude-Angle29/1
  [Vabc_30] -> Complex to Magnitude-Angle30/1
  [Vabc_26] -> Complex to Magnitude-Angle28/1
  [Vabc_27] -> Complex to Magnitude-Angle26/1
  [Vabc_28] -> Complex to Magnitude-Angle27/1
  Complex to Magnitude-Angle28/1 -> Display33/1, Scope28/1
  Complex to Magnitude-Angle27/1 -> Display35/1, Scope27/1
  Complex to Magnitude-Angle29/1 -> Display36/1, Scope29/1
  Complex to Magnitude-Angle30/1 -> Display32/1, Scope30/1
  Complex to Magnitude-Angle26/1 -> Display34/1, Scope26/1
  [Vabc_36] -> Complex to Magnitude-Angle34/1
  [Vabc_37] -> Complex to Magnitude-Angle35/1
  [Vabc_38] -> Complex to Magnitude-Angle31/1
  [Vabc_39] -> Complex to Magnitude-Angle32/1
  Complex to Magnitude-Angle34/1 -> Display37/1, Scope34/1
  Complex to Magnitude-Angle31/1 -> Display39/1, Scope31/1
  Complex to Magnitude-Angle32/1 -> Display40/1, Scope32/1
  Complex to Magnitude-Angle35/1 -> Display38/1, Scope35/1

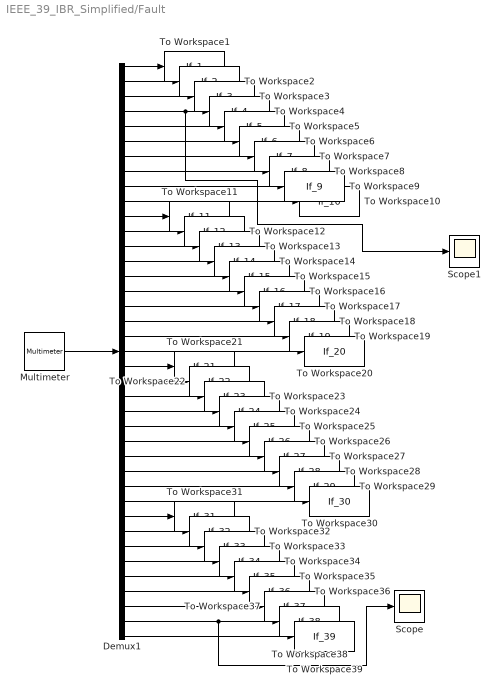
== system IEEE_39_IBR_Simplified/Fault ==
  Demux1 : Demux  Outputs=39
  Multimeter : spsMultimeterLib/Multimeter  L=234  sel=[142 229 232 169 172 175 178 181 184 145 148 151 154 157 187 190 223 226 193 196 199 202 205 208 118 121 124 127 130 133 160 163 211 214 217 220 136 139 166]  yselected={}  Gain=[1 1 1 1 1 1 1 1 1 1 1 1 1 1 1 1 1 1 1 1 1 1 1 1 1 1 1 1 1 1 1 1 1 1 1 1 1 1 1]  OutputType=Magnitude  PlotAtSimulationStop=off  PhasorSimulation=off
  Scope : Scope
  Scope1 : Scope
  To Workspace1 : ToWorkspace  VariableName=If_1  SaveFormat=Timeseries  SampleTime=-1
  To Workspace10 : ToWorkspace  VariableName=If_10  SaveFormat=Timeseries  SampleTime=-1
  To Workspace11 : ToWorkspace  VariableName=If_11  SaveFormat=Timeseries  SampleTime=-1
  To Workspace12 : ToWorkspace  VariableName=If_12  SaveFormat=Timeseries  SampleTime=-1
  To Workspace13 : ToWorkspace  VariableName=If_13  SaveFormat=Timeseries  SampleTime=-1
  To Workspace14 : ToWorkspace  VariableName=If_14  SaveFormat=Timeseries  SampleTime=-1
  To Workspace15 : ToWorkspace  VariableName=If_15  SaveFormat=Timeseries  SampleTime=-1
  To Workspace16 : ToWorkspace  VariableName=If_16  SaveFormat=Timeseries  SampleTime=-1
  To Workspace17 : ToWorkspace  VariableName=If_17  SaveFormat=Timeseries  SampleTime=-1
  To Workspace18 : ToWorkspace  VariableName=If_18  SaveFormat=Timeseries  SampleTime=-1
  To Workspace19 : ToWorkspace  VariableName=If_19  SaveFormat=Timeseries  SampleTime=-1
  To Workspace2 : ToWorkspace  VariableName=If_2  SaveFormat=Timeseries  SampleTime=-1
  To Workspace20 : ToWorkspace  VariableName=If_20  SaveFormat=Timeseries  SampleTime=-1
  To Workspace21 : ToWorkspace  VariableName=If_21  SaveFormat=Timeseries  SampleTime=-1
  To Workspace22 : ToWorkspace  VariableName=If_22  SaveFormat=Timeseries  SampleTime=-1
  To Workspace23 : ToWorkspace  VariableName=If_23  SaveFormat=Timeseries  SampleTime=-1
  To Workspace24 : ToWorkspace  VariableName=If_24  SaveFormat=Timeseries  SampleTime=-1
  To Workspace25 : ToWorkspace  VariableName=If_25  SaveFormat=Timeseries  SampleTime=-1
  To Workspace26 : ToWorkspace  VariableName=If_26  SaveFormat=Timeseries  SampleTime=-1
  To Workspace27 : ToWorkspace  VariableName=If_27  SaveFormat=Timeseries  SampleTime=-1
  To Workspace28 : ToWorkspace  VariableName=If_28  SaveFormat=Timeseries  SampleTime=-1
  To Workspace29 : ToWorkspace  VariableName=If_29  SaveFormat=Timeseries  SampleTime=-1
  To Workspace3 : ToWorkspace  VariableName=If_3  SaveFormat=Timeseries  SampleTime=-1
  To Workspace30 : ToWorkspace  VariableName=If_30  SaveFormat=Timeseries  SampleTime=-1
  To Workspace31 : ToWorkspace  VariableName=If_31  SaveFormat=Timeseries  SampleTime=-1
  To Workspace32 : ToWorkspace  VariableName=If_32  SaveFormat=Timeseries  SampleTime=-1
  To Workspace33 : ToWorkspace  VariableName=If_33  SaveFormat=Timeseries  SampleTime=-1
  To Workspace34 : ToWorkspace  VariableName=If_34  SaveFormat=Timeseries  SampleTime=-1
  To Workspace35 : ToWorkspace  VariableName=If_35  SaveFormat=Timeseries  SampleTime=-1
  To Workspace36 : ToWorkspace  VariableName=If_36  SaveFormat=Timeseries  SampleTime=-1
  To Workspace37 : ToWorkspace  VariableName=If_37  SaveFormat=Timeseries  SampleTime=-1
  To Workspace38 : ToWorkspace  VariableName=If_38  SaveFormat=Timeseries  SampleTime=-1
  To Workspace39 : ToWorkspace  VariableName=If_39  SaveFormat=Timeseries  SampleTime=-1
  To Workspace4 : ToWorkspace  VariableName=If_4  SaveFormat=Timeseries  SampleTime=-1
  To Workspace5 : ToWorkspace  VariableName=If_5  SaveFormat=Timeseries  SampleTime=-1
  To Workspace6 : ToWorkspace  VariableName=If_6  SaveFormat=Timeseries  SampleTime=-1
  To Workspace7 : ToWorkspace  VariableName=If_7  SaveFormat=Timeseries  SampleTime=-1
  To Workspace8 : ToWorkspace  VariableName=If_8  SaveFormat=Timeseries  SampleTime=-1
  To Workspace9 : ToWorkspace  VariableName=If_9  SaveFormat=Timeseries  SampleTime=-1
  wires:
  Multimeter/1 -> Demux1/1
  Demux1/1 -> To Workspace1/1
  Demux1/2 -> To Workspace2/1
  Demux1/3 -> To Workspace3/1
  Demux1/4 -> Scope1/1, To Workspace4/1
  Demux1/5 -> To Workspace5/1
  Demux1/6 -> To Workspace6/1
  Demux1/7 -> To Workspace7/1
  Demux1/8 -> To Workspace8/1
  Demux1/9 -> To Workspace9/1
  Demux1/10 -> To Workspace10/1
  Demux1/11 -> To Workspace11/1
  Demux1/12 -> To Workspace12/1
  Demux1/13 -> To Workspace13/1
  Demux1/14 -> To Workspace14/1
  Demux1/15 -> To Workspace15/1
  Demux1/16 -> To Workspace16/1
  Demux1/17 -> To Workspace17/1
  Demux1/18 -> To Workspace18/1
  Demux1/19 -> To Workspace19/1
  Demux1/20 -> To Workspace20/1
  Demux1/21 -> To Workspace21/1
  Demux1/22 -> To Workspace22/1
  Demux1/23 -> To Workspace23/1
  Demux1/24 -> To Workspace24/1
  Demux1/25 -> To Workspace25/1
  Demux1/26 -> To Workspace26/1
  Demux1/27 -> To Workspace27/1
  Demux1/28 -> To Workspace28/1
  Demux1/29 -> To Workspace29/1
  Demux1/30 -> To Workspace30/1
  Demux1/31 -> To Workspace31/1
  Demux1/32 -> To Workspace32/1
  Demux1/33 -> To Workspace33/1
  Demux1/34 -> To Workspace34/1
  Demux1/35 -> To Workspace35/1
  Demux1/36 -> To Workspace36/1
  Demux1/37 -> To Workspace37/1
  Demux1/38 -> Scope/1, To Workspace38/1
  Demux1/39 -> To Workspace39/1

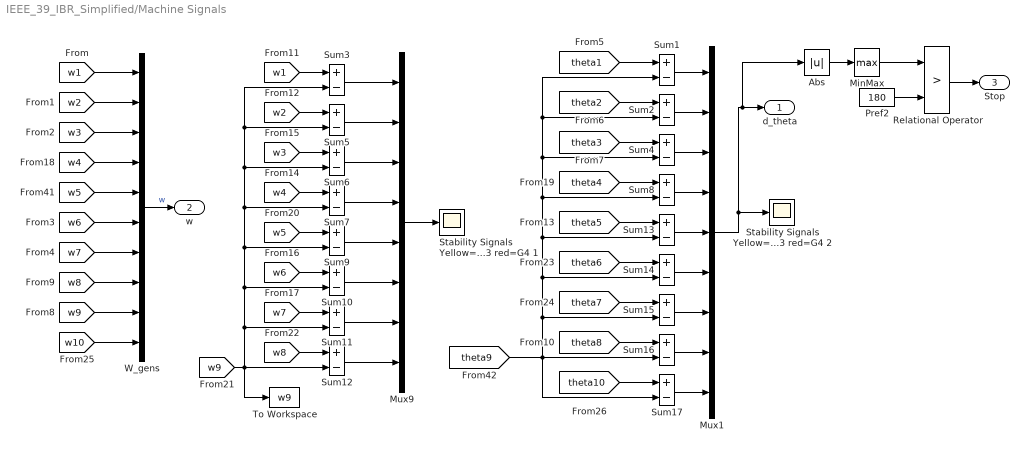
== system IEEE_39_IBR_Simplified/Machine Signals ==
  Abs : Abs
  MinMax : MinMax  Function=max  InputSameDT=on  SaturateOnIntegerOverflow=on
  Mux1 : Mux  Inputs=9
  Mux9 : Mux  Inputs=8
  Pref2 : Constant  Value=180
  Relational Operator : RelationalOperator  Operator=>
  Stability Signals Yellow=G1 mag=G2 cyan=G3 red=G4 1 : Scope
  Stability Signals Yellow=G1 mag=G2 cyan=G3 red=G4 2 : Scope
  Sum{1..17} (17 alike) : Sum  Inputs=+-  InputSameDT=on  SaturateOnIntegerOverflow=on  OutDataTypeStr=Inherit: Same as first input
  To Workspace : ToWorkspace  VariableName=w9  SaveFormat=Timeseries  SampleTime=-1
  W_gens : Mux  Inputs=10
  d_theta : Outport  VectorParamsAs1DForOutWhenUnconnected=off
  w : Outport  Port=2  VectorParamsAs1DForOutWhenUnconnected=off
  Stop : Outport  Port=3  VectorParamsAs1DForOutWhenUnconnected=off
  wires:
  Abs/1 -> MinMax/1
  Pref2/1 -> Relational Operator/2
  MinMax/1 -> Relational Operator/1
  W_gens/1 -> w/1  "w"
  Relational Operator/1 -> Stop/1
  Mux9/1 -> Stability Signals Yellow=G1 mag=G2 cyan=G3 red=G4 1/1
  [w1] -> W_gens/1
  [w2] -> W_gens/2
  [w4] -> W_gens/4
  [w3] -> W_gens/3
  [w5] -> W_gens/5
  [w9] -> W_gens/9
  [w8] -> W_gens/8
  [w7] -> W_gens/7
  [w6] -> W_gens/6
  [w1] -> Sum3/1
  [w2] -> Sum5/1
  [w4] -> Sum7/1
  [w3] -> Sum6/1
  [w5] -> Sum9/1
  [w9] -> To Workspace/1, Sum11/2, Sum10/2, Sum9/2, Sum7/2, Sum6/2, Sum5/2, Sum3/2, Sum12/2
  [w8] -> Sum12/1
  [w7] -> Sum11/1
  [w6] -> Sum10/1
  Sum7/1 -> Mux9/4
  Sum6/1 -> Mux9/3
  Sum5/1 -> Mux9/2
  Sum3/1 -> Mux9/1
  Sum10/1 -> Mux9/6
  Sum9/1 -> Mux9/5
  Sum11/1 -> Mux9/7
  Sum12/1 -> Mux9/8
  [theta8] -> Sum16/1
  [theta1] -> Sum1/1
  [theta2] -> Sum2/1
  [theta3] -> Sum4/1
  [theta4] -> Sum8/1
  [theta5] -> Sum13/1
  [theta6] -> Sum14/1
  [theta7] -> Sum15/1
  Sum2/1 -> Mux1/2
  Sum1/1 -> Mux1/1
  Sum4/1 -> Mux1/3
  Sum8/1 -> Mux1/4
  Sum13/1 -> Mux1/5
  Sum14/1 -> Mux1/6
  Sum15/1 -> Mux1/7
  Sum16/1 -> Mux1/8
  Mux1/1 -> Abs/1, d_theta/1, Stability Signals Yellow=G1 mag=G2 cyan=G3 red=G4 2/1
  [w10] -> W_gens/10
  [theta10] -> Sum17/1
  [theta9] -> Sum17/2, Sum15/2, Sum14/2, Sum4/2, Sum1/2, Sum2/2, Sum8/2, Sum13/2, Sum16/2
  Sum17/1 -> Mux1/9

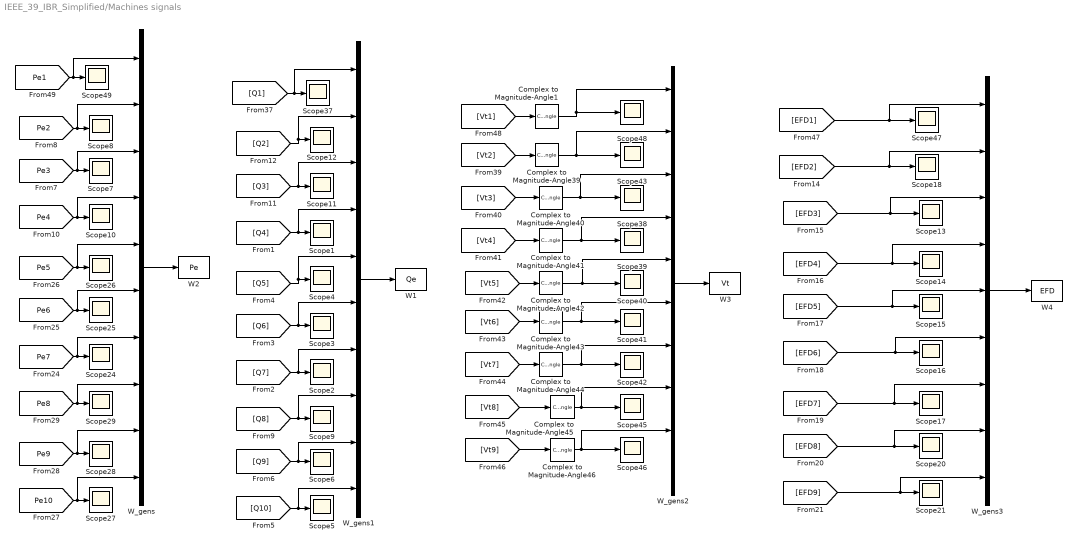
== system IEEE_39_IBR_Simplified/Machines signals ==
  Complex to Magnitude-Angle{1,39..46} (9 alike) : ComplexToMagnitudeAngle  Output=Magnitude
  Scope{1..18,20..21,24..29,37..43,45..49} (38 alike) : Scope
  W1 : ToWorkspace  VariableName=Qe  SampleTime=-1
  W2 : ToWorkspace  VariableName=Pe  SampleTime=-1
  W3 : ToWorkspace  VariableName=Vt  SampleTime=-1
  W4 : ToWorkspace  VariableName=EFD  SampleTime=-1
  W_gens : Mux  Inputs=10
  W_gens1 : Mux  Inputs=10
  W_gens2 : Mux  Inputs=10
  W_gens3 : Mux  Inputs=9
  wires:
  [Pe3] -> W_gens/3, Scope7/1
  [Pe2] -> W_gens/2, Scope8/1
  [Vt2] -> Complex to Magnitude-Angle39/1
  Complex to Magnitude-Angle39/1 -> Scope43/1, W_gens2/2
  [Vt3] -> Complex to Magnitude-Angle40/1
  Complex to Magnitude-Angle40/1 -> Scope38/1, W_gens2/3
  [Vt4] -> Complex to Magnitude-Angle41/1
  Complex to Magnitude-Angle41/1 -> Scope39/1, W_gens2/4
  [Vt5] -> Complex to Magnitude-Angle42/1
  Complex to Magnitude-Angle42/1 -> Scope40/1, W_gens2/5
  [Vt6] -> Complex to Magnitude-Angle43/1
  Complex to Magnitude-Angle43/1 -> W_gens2/6, Scope41/1
  [Vt7] -> Complex to Magnitude-Angle44/1
  Complex to Magnitude-Angle44/1 -> Scope42/1, W_gens2/7
  [Vt8] -> Complex to Magnitude-Angle45/1
  Complex to Magnitude-Angle45/1 -> Scope45/1, W_gens2/8
  [Vt9] -> Complex to Magnitude-Angle46/1
  Complex to Magnitude-Angle46/1 -> W_gens2/9, Scope46/1
  [Pe6] -> W_gens/6, Scope25/1
  [Pe5] -> W_gens/5, Scope26/1
  [Pe7] -> W_gens/7, Scope24/1
  [Pe9] -> W_gens/9, Scope28/1
  [Pe8] -> W_gens/8, Scope29/1
  [Pe10] -> W_gens/10, Scope27/1
  [Q3] -> W_gens1/3, Scope11/1
  [Q2] -> W_gens1/2, Scope12/1
  [Q4] -> W_gens1/4, Scope1/1
  [Q6] -> W_gens1/6, Scope3/1
  [Q5] -> W_gens1/5, Scope4/1
  [Q7] -> W_gens1/7, Scope2/1
  [Q9] -> W_gens1/9, Scope6/1
  [Q8] -> W_gens1/8, Scope9/1
  [Q10] -> W_gens1/10, Scope5/1
  [EFD2] -> W_gens3/2, Scope18/1
  [EFD3] -> Scope13/1, W_gens3/3
  [EFD4] -> W_gens3/4, Scope14/1
  [EFD5] -> W_gens3/5, Scope15/1
  [EFD6] -> W_gens3/6, Scope16/1
  [EFD7] -> W_gens3/7, Scope17/1
  [EFD8] -> W_gens3/8, Scope20/1
  [EFD9] -> Scope21/1, W_gens3/9
  [Pe4] -> W_gens/4, Scope10/1
  [Pe1] -> W_gens/1, Scope49/1
  Complex to Magnitude-Angle1/1 -> W_gens2/1, Scope48/1
  [Q1] -> W_gens1/1, Scope37/1
  [EFD1] -> W_gens3/1, Scope47/1
  [Vt1] -> Complex to Magnitude-Angle1/1
  W_gens/1 -> W2/1
  W_gens1/1 -> W1/1
  W_gens2/1 -> W3/1
  W_gens3/1 -> W4/1

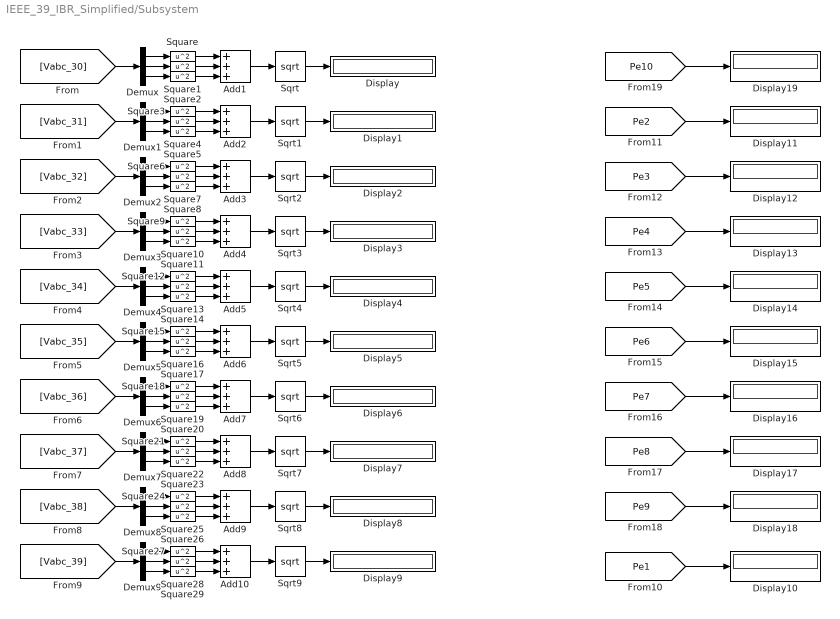
== system IEEE_39_IBR_Simplified/Subsystem ==
  Add{1..10} (10 alike) : Sum  Inputs=+++
  Demux{,1..9} (10 alike) : Demux  Outputs=3
  Display{,1..19} (20 alike) : Display
  Sqrt{,1..9} (10 alike) : Sqrt
  Square{,1..29} (30 alike) : Math  Operator=square
  wires:
  [Pe1] -> Display10/1
  [Pe2] -> Display11/1
  [Pe3] -> Display12/1
  [Pe4] -> Display13/1
  [Pe5] -> Display14/1
  [Pe6] -> Display15/1
  [Pe7] -> Display16/1
  [Pe8] -> Display17/1
  [Pe9] -> Display18/1
  [Pe10] -> Display19/1
  [Vabc_30] -> Demux/1
  Demux/1 -> Square/1
  Square/1 -> Add1/1
  Demux/2 -> Square1/1
  Square1/1 -> Add1/2
  Demux/3 -> Square2/1
  Square2/1 -> Add1/3
  Square4/1 -> Add2/2
  Demux1/2 -> Square4/1
  Square3/1 -> Add2/1
  [Vabc_31] -> Demux1/1
  Square5/1 -> Add2/3
  Demux1/3 -> Square5/1
  Square7/1 -> Add3/2
  Demux2/2 -> Square7/1
  Square6/1 -> Add3/1
  [Vabc_32] -> Demux2/1
  Square8/1 -> Add3/3
  Demux2/3 -> Square8/1
  Demux2/1 -> Square6/1
  Square10/1 -> Add4/2
  Demux3/2 -> Square10/1
  Square9/1 -> Add4/1
  [Vabc_33] -> Demux3/1
  Square11/1 -> Add4/3
  Demux3/3 -> Square11/1
  Demux3/1 -> Square9/1
  Square13/1 -> Add5/2
  Demux4/2 -> Square13/1
  Square12/1 -> Add5/1
  [Vabc_34] -> Demux4/1
  Square14/1 -> Add5/3
  Demux4/3 -> Square14/1
  Demux4/1 -> Square12/1
  Square16/1 -> Add6/2
  Demux5/2 -> Square16/1
  Square15/1 -> Add6/1
  [Vabc_35] -> Demux5/1
  Square17/1 -> Add6/3
  Demux5/3 -> Square17/1
  Demux5/1 -> Square15/1
  Demux6/1 -> Square18/1
  Demux6/2 -> Square19/1
  Square20/1 -> Add7/3
  Demux6/3 -> Square20/1
  Square19/1 -> Add7/2
  Square18/1 -> Add7/1
  [Vabc_36] -> Demux6/1
  Demux7/1 -> Square21/1
  Demux7/2 -> Square22/1
  Square23/1 -> Add8/3
  Demux7/3 -> Square23/1
  Square22/1 -> Add8/2
  Square21/1 -> Add8/1
  [Vabc_37] -> Demux7/1
  Demux8/1 -> Square24/1
  Demux8/2 -> Square25/1
  Square26/1 -> Add9/3
  Demux8/3 -> Square26/1
  Square25/1 -> Add9/2
  Square24/1 -> Add9/1
  [Vabc_38] -> Demux8/1
  Demux9/1 -> Square27/1
  Demux9/2 -> Square28/1
  Square29/1 -> Add10/3
  Demux9/3 -> Square29/1
  Square28/1 -> Add10/2
  Square27/1 -> Add10/1
  [Vabc_39] -> Demux9/1
  Add1/1 -> Sqrt/1
  Sqrt/1 -> Display/1
  Sqrt1/1 -> Display1/1
  Add2/1 -> Sqrt1/1
  Sqrt2/1 -> Display2/1
  Add3/1 -> Sqrt2/1
  Sqrt3/1 -> Display3/1
  Add4/1 -> Sqrt3/1
  Sqrt4/1 -> Display4/1
  Add5/1 -> Sqrt4/1
  Sqrt5/1 -> Display5/1
  Add6/1 -> Sqrt5/1
  Sqrt6/1 -> Display6/1
  Add7/1 -> Sqrt6/1
  Sqrt7/1 -> Display7/1
  Add8/1 -> Sqrt7/1
  Sqrt8/1 -> Display8/1
  Add9/1 -> Sqrt8/1
  Sqrt9/1 -> Display9/1
  Add10/1 -> Sqrt9/1
  Demux1/1 -> Square3/1

== system IEEE_39_IBR_Simplified/System Data ==
  ->pu : Gain  Gain=1/(230e3/sqrt(3)*sqrt(2))  SaturateOnIntegerOverflow=on  OutDataTypeStr=Inherit: Same as input  ParamDataTypeStr=Inherit: Same as input
  Complex to Magnitude-Angle : ComplexToMagnitudeAngle  Output=Magnitude
  Complex to Magnitude-Angle1 : ComplexToMagnitudeAngle  Output=Magnitude
  Mux : Mux  Inputs=2
  P34 : Gain  Gain=1e-6  SaturateOnIntegerOverflow=on  OutDataTypeStr=Inherit: Same as input  ParamDataTypeStr=Inherit: Same as input
  Sequence Analyzer : spsSequenceAnalyzerLib/Sequence Analyzer  Freq=60  n=1  seq=Positive Negative Zero  InInit=[1, 0]  Ts=0
      settings: LibrarySourceBlock=sps_lib/Sensors and Measurements/Sequence Analyzer
  Sequence Analyzer1 : spsSequenceAnalyzerLib/Sequence Analyzer  Freq=60  n=1  seq=Positive Negative Zero  InInit=[1, 0]  Ts=0
      settings: LibrarySourceBlock=sps_lib/Sensors and Measurements/Sequence Analyzer
  Terminator1 : Terminator
  Terminator2 : Terminator
  Terminator3 : Terminator
  Three-Phase Power Measurement : eePowerMeasurement/Power Measurement (Three-Phase)  LabelModeActiveChoice=Continuous  F=60  K=[0 1 2 3]  Seq=Positive  Ts=0
  Vabc_B3 : Scope
  Vabc_B4 : Scope
  W2 : ToWorkspace  VariableName=P21  SampleTime=-1
  Vps : Outport  VectorParamsAs1DForOutWhenUnconnected=off
  p34 : Outport  Port=2  VectorParamsAs1DForOutWhenUnconnected=off
  wires:
  [Vabc_B4] -> Three-Phase Power Measurement/1, Sequence Analyzer/1, Complex to Magnitude-Angle/1
  [Vabc_B3] -> Sequence Analyzer1/1, Complex to Magnitude-Angle1/1
  Sequence Analyzer/2 -> Terminator1/1
  Sequence Analyzer1/2 -> Terminator2/1
  Sequence Analyzer1/1 -> Mux/2
  [Iabc_B4] -> Three-Phase Power Measurement/2
  ->pu/1 -> Vps/1
  Sequence Analyzer/1 -> Mux/1
  Mux/1 -> ->pu/1
  P34/1 -> W2/1, p34/1
  Complex to Magnitude-Angle/1 -> Vabc_B4/1
  Complex to Magnitude-Angle1/1 -> Vabc_B3/1
  Three-Phase Power Measurement/1 -> P34/1
  Three-Phase Power Measurement/2 -> Terminator3/1

== system IEEE_39_IBR_Simplified/A1/G10 ==
  Controllers : Subsystem
  Simplified Synchronous Machine pu Units : spsSimplifiedSynchronousMachinepuUnitsLib/Simplified Synchronous Machine pu Units  ConnectionType=3-wire Y  MechanicalLoad=Mechanical power Pm  MeasurementBus=off  NominalParameters="[ Pn_sm(10)*1e6  Un_sm(10)*1e3  fn_sm(10) ]"  Mechanical=[ H_sm(10) Kd_sm(10) p]  InternalRL="[rs  xd]"  InitialConditions=[dw0_sm theta0_sm ia0_sm ib0_sm ic0_sm pha0_sm phb0_sm phc0_sm]  IterativeDiscreteModel=Trapezoidal non iterative  TsBlock=-1  TsPowergui=0  LoadFlowParameters=[1,0,0,0,0]  Units=0  BusType=PV  Pref=0  Qref=0  Qmin=-inf  Qmax=+inf  PLF=0  QLF=0
      settings: LibrarySourceBlock=|
      | sps_lib/Electrical Machines/Simplified Synchronous
      | Machine pu Units
  A : PMIOPort  Side=Left
  B : PMIOPort  Port=2  Side=Left
  C : PMIOPort  Port=3  Side=Left
  wires:
  Controllers/1(Pm) -> Simplified Synchronous Machine pu Units/1
  Simplified Synchronous Machine pu Units/1 -> Controllers/1(m)
  Controllers/2(Vref) -> Simplified Synchronous Machine pu Units/2
  connections:
  Simplified Synchronous Machine pu Units/RConn2 -- B/RConn1
  Simplified Synchronous Machine pu Units/RConn3 -- C/RConn1
  Simplified Synchronous Machine pu Units/RConn1 -- A/RConn1

== system IEEE_39_IBR_Simplified/A1/G8 ==
  Controllers : Subsystem
  Simplified Synchronous Machine pu Units : spsSimplifiedSynchronousMachinepuUnitsLib/Simplified Synchronous Machine pu Units  ConnectionType=3-wire Y  MechanicalLoad=Mechanical power Pm  MeasurementBus=off  NominalParameters="[ Pn_sm(8)*1e6  Un_sm(8)*1e3  fn_sm(8) ]"  Mechanical=[ H_sm(8) Kd_sm(8) p]  InternalRL="[rs  xd]"  InitialConditions=[dw0_sm theta0_sm ia0_sm ib0_sm ic0_sm pha0_sm phb0_sm phc0_sm]  IterativeDiscreteModel=Trapezoidal non iterative  TsBlock=-1  TsPowergui=0  LoadFlowParameters=[1,0,0,0,0]  Units=0  BusType=PV  Pref=0  Qref=0  Qmin=-inf  Qmax=+inf  PLF=0  QLF=0
      settings: LibrarySourceBlock=|
      | sps_lib/Electrical Machines/Simplified Synchronous
      | Machine pu Units
  A : PMIOPort  Side=Left
  B : PMIOPort  Port=2  Side=Left
  C : PMIOPort  Port=3  Side=Left
  wires:
  Controllers/1(Pm) -> Simplified Synchronous Machine pu Units/1
  Simplified Synchronous Machine pu Units/1 -> Controllers/1(m)
  Controllers/2(Vref) -> Simplified Synchronous Machine pu Units/2
  connections:
  Simplified Synchronous Machine pu Units/RConn2 -- B/RConn1
  Simplified Synchronous Machine pu Units/RConn3 -- C/RConn1
  Simplified Synchronous Machine pu Units/RConn1 -- A/RConn1

== system IEEE_39_IBR_Simplified/A1/G9 ==
  Controllers : Subsystem
  Simplified Synchronous Machine pu Units : spsSimplifiedSynchronousMachinepuUnitsLib/Simplified Synchronous Machine pu Units  ConnectionType=3-wire Y  MechanicalLoad=Mechanical power Pm  MeasurementBus=off  NominalParameters="[ Pn_sm(9)*1e6  Un_sm(9)*1e3  fn_sm(9) ]"  Mechanical=[ H_sm(9) Kd_sm(9) p]  InternalRL="[rs  xd]"  InitialConditions=[dw0_sm theta0_sm ia0_sm ib0_sm ic0_sm pha0_sm phb0_sm phc0_sm]  IterativeDiscreteModel=Trapezoidal non iterative  TsBlock=-1  TsPowergui=0  LoadFlowParameters=[1,0,0,0,0]  Units=0  BusType=PV  Pref=0  Qref=0  Qmin=-inf  Qmax=+inf  PLF=0  QLF=0
      settings: LibrarySourceBlock=|
      | sps_lib/Electrical Machines/Simplified Synchronous
      | Machine pu Units
  A : PMIOPort  Side=Left
  B : PMIOPort  Port=2  Side=Left
  C : PMIOPort  Port=3  Side=Left
  wires:
  Controllers/1(Pm) -> Simplified Synchronous Machine pu Units/1
  Simplified Synchronous Machine pu Units/1 -> Controllers/1(m)
  Controllers/2(Vref) -> Simplified Synchronous Machine pu Units/2
  connections:
  Simplified Synchronous Machine pu Units/RConn2 -- B/RConn1
  Simplified Synchronous Machine pu Units/RConn3 -- C/RConn1
  Simplified Synchronous Machine pu Units/RConn1 -- A/RConn1
